simulink model "PF_ParallelHybrid_AllElectric"  (R2021b)
settings: Solver=FixedStepAuto  StartTime=0.0  StopTime=10  FixedStep=0.02  RelTol=1e-3
libraries: Lib_EMTAT x6, slpidlib x1
settings Model: Creator=sbianco1  LastModifiedBy=sbianco1
settings SolverCC: AlgebraicLoopSolver=TrustRegion
settings DebuggingCC: SFMachineParentedDataDiag=warning

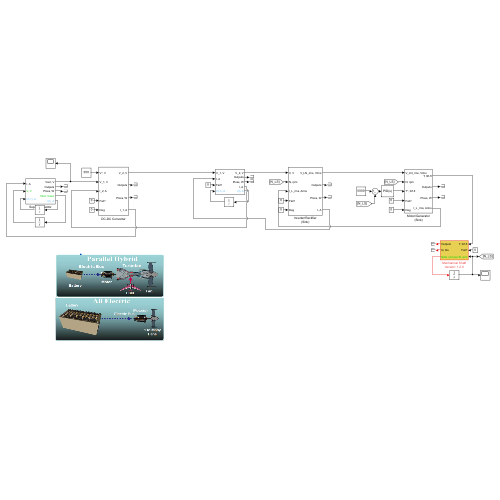
[thumbnail: Simulink's stored preview of the top-level diagram]
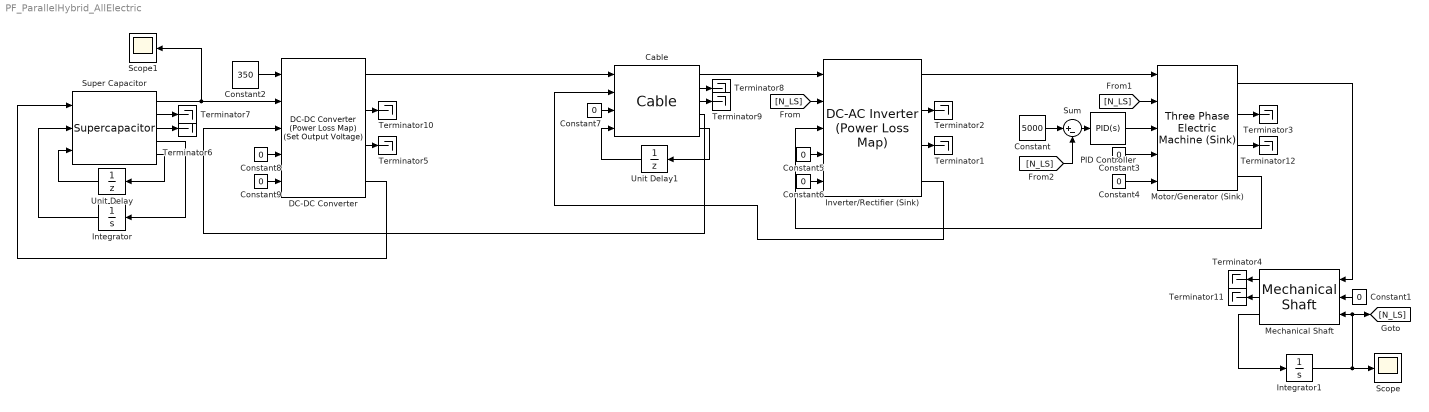
== system PF_ParallelHybrid_AllElectric ==
  Cable : Lib_EMTAT/Components/Power Flow/Cable  R=0.2
  Constant : Constant  Value=5000
  Constant{1,3..9} (8 alike) : Constant  Value=0
  Constant2 : Constant  Value=350
  DC-DC Converter : Lib_EMTAT/Components/Power Flow/DC-DC Converter (Power Loss Map) (Set Output Voltage)  X_Vin_VoltageVec_M=[0 100 1000 5000]  Y_Iout_CurrentVec_M=[0 10 100 150]  T_C_PlossArray_M=100*ones(4,4)  FM=0  Plosslim=0
  Integrator : Integrator  InitialCondition=150
  Integrator1 : Integrator  InitialCondition=5000
  Inverter/Rectifier (Sink) : Lib_EMTAT/Components/Power Flow/DC-AC Inverter (Power Loss Map)  X_C_VoltageInVec_M=[0 1000]  Y_C_RMSCurrentOutVec_M=[0 1000]  T_C_PowLossArray_M=100*ones(2)  K_e=0.0503  FM=0  Plosslim=0
  Mechanical Shaft : Lib_EMTAT/Components/Power Flow/Mechanical Shaft  J=0.01  B=0.001
      settings: AttributesFormatString=|
      | Mechanical Shaft
      | Version: %<LibraryVersion>
  Motor/Generator (Sink) : Lib_EMTAT/Components/Power Flow/Three Phase Electric Machine (Sink)  X_C_SpeedVec_M=[0 100 1000 5000]  Y_C_TorqueVec_M=[0 10 100 150]  T_C_EffArray_M=0.99*ones(4,4)  FM=0
  PID Controller : slpidlib/PID Controller  Controller=PID  Form=Parallel  TimeDomain=Continuous-time  UseExternalTs=off  SampleTime=-1  IntegratorMethod=Forward Euler  FilterMethod=Forward Euler  ControllerParametersSource=internal  P=0.01  I=0.01  D=0  N=100  UseFilter=on  TunerSelectOption=Transfer Function Based (PID Tuner App)  InitialConditionSource=internal  InitialConditionForIntegrator=0  InitialConditionForFilter=0  DifferentiatorICPrevScaledInput=0  ExternalReset=none  TrackingMode=off  Kt=1  LimitOutput=off  SatLimitsSource=internal  UpperSaturationLimit=inf  LowerSaturationLimit=-inf  LinearizeAsGain=on  AntiWindupMode=none  Kb=1  POutMin=[]  POutMax=[]  IOutMin=[]  IOutMax=[]  DOutMin=[]  DOutMax=[]  NOutMin=[]  NOutMax=[]  SumOutMin=[]  SumOutMax=[]  SaturationOutMin=[]  SaturationOutMax=[]  PParamMin=[]  PParamMax=[]  IParamMin=[]  IParamMax=[]  DParamMin=[]  DParamMax=[]  NParamMin=[]  NParamMax=[]  KbParamMin=[]  KbParamMax=[]  KtParamMin=[]  KtParamMax=[]  KbOutMin=[]  KbOutMax=[]  KtOutMin=[]  KtOutMax=[]  IntegratorOutMin=[]  IntegratorOutMax=[]  FilterOutMin=[]  FilterOutMax=[]  SumI1OutMin=[]  SumI1OutMax=[]  SumI2OutMin=[]  SumI2OutMax=[]  SumI3OutMin=[]  SumI3OutMax=[]  SumI4OutMin=[]  SumI4OutMax=[]  SumDOutMin=[]  SumDOutMax=[]  DifferentiatorOutMin=[]  DifferentiatorOutMax=[]  FilterDiffOutCoefMin=[]  FilterDiffOutCoefMax=[]  ReciprocalOutMin=[]  ReciprocalOutMax=[]  SumDenOutMin=[]  SumDenOutMax=[]  SumNumOutMin=[]  SumNumOutMax=[]  DivideOutMin=[]  DivideOutMax=[]  UdiffTsProdOutMin=[]  UdiffTsProdOutMax=[]  NTsProdOutMin=[]  NTsProdOutMax=[]  UintegralTsProdOutMin=[]  UintegralTsProdOutMax=[]  UngainTsProdOutMin=[]  UngainTsProdOutMax=[]  IntegratorContinuousStateAttributes=''  IntegratorStateMustResolveToSignalObject=off  IntegratorRTWStateStorageClass=Auto  FilterContinuousStateAttributes=''  FilterStateMustResolveToSignalObject=off  FilterRTWStateStorageClass=Auto  ParallelPVariant=InternalParameters  IdealPVariant=Disabled  IVariant=InternalParameters  DVariant=InternalParameters  IntegratorVariant=Continuous  SatVariant=Disabled  AWVariant=Passthrough  PCopyVariant=Disabled  TRVariant=Disabled  FdbkBlocksVariant=Forward  IdealPFdbkVariant=Disabled  SatFdbkVariant=Disabled  DerivativeFilterVariant=ContFilter  NVariant=InternalParameters  NCopyVariant=Disabled  FilterICVariant=InternalICsFilter  IntegratorICVariant=InternalICs  ExternalResetVariant=Disabled  TRSumVariant=Passthrough  SumFdbkVariant=Disabled  SumVariant=Sum_PID  TsampFilterVariant=InternalTs  TsampNgainVariant=Passthrough  TsampIntegralVariant=Passthrough  ExternalSaturationOutDataTypeStr=Inherit: Same as second input
  Scope : Scope
  Scope1 : Scope
  Sum : Sum  Inputs=|+-
  Super Capacitor : Lib_EMTAT/Components/Power Flow/Supercapacitor  C=130  ESR=0.02  TSE=200  BlkNm=double(gcb)
  Terminator{1..12} (12 alike) : Terminator
  Unit Delay : UnitDelay  SampleTime=-1  HasFrameUpgradeWarning=on
  Unit Delay1 : UnitDelay  SampleTime=-1  HasFrameUpgradeWarning=on
  wires:
  Inverter/Rectifier (Sink)/1 -> Motor/Generator (Sink)/1
  Constant2/1 -> DC-DC Converter/1
  Super Capacitor/1 -> Scope1/1, DC-DC Converter/2
  Cable/1 -> Inverter/Rectifier (Sink)/1
  Inverter/Rectifier (Sink)/4 -> Cable/2
  Motor/Generator (Sink)/4 -> Inverter/Rectifier (Sink)/3
  [N_LS] -> Inverter/Rectifier (Sink)/2
  [N_LS] -> Motor/Generator (Sink)/2
  Motor/Generator (Sink)/1 -> Mechanical Shaft/1
  Inverter/Rectifier (Sink)/3 -> Terminator1/1
  Inverter/Rectifier (Sink)/2 -> Terminator2/1
  Motor/Generator (Sink)/2 -> Terminator3/1
  DC-DC Converter/4 -> Super Capacitor/1
  Cable/4 -> DC-DC Converter/3
  Super Capacitor/3 -> Terminator6/1
  Super Capacitor/2 -> Terminator7/1
  DC-DC Converter/1 -> Cable/1
  Cable/2 -> Terminator8/1
  Cable/3 -> Terminator9/1
  [N_LS] -> Sum/2
  Sum/1 -> PID Controller/1
  Constant/1 -> Sum/1
  PID Controller/1 -> Motor/Generator (Sink)/3
  DC-DC Converter/3 -> Terminator5/1
  DC-DC Converter/2 -> Terminator10/1
  Super Capacitor/5 -> Unit Delay/1
  Unit Delay/1 -> Super Capacitor/3
  Integrator/1 -> Super Capacitor/2
  Super Capacitor/4 -> Integrator/1
  Cable/5 -> Unit Delay1/1
  Unit Delay1/1 -> Cable/4
  Integrator1/1 -> Scope/1, [N_LS], Mechanical Shaft/3
  Constant1/1 -> Mechanical Shaft/2
  Motor/Generator (Sink)/3 -> Terminator12/1
  Constant3/1 -> Motor/Generator (Sink)/4
  Constant4/1 -> Motor/Generator (Sink)/5
  Constant5/1 -> Inverter/Rectifier (Sink)/4
  Constant6/1 -> Inverter/Rectifier (Sink)/5
  Constant7/1 -> Cable/3
  Constant8/1 -> DC-DC Converter/4
  Constant9/1 -> DC-DC Converter/5
  Mechanical Shaft/1 -> Terminator4/1
  Mechanical Shaft/2 -> Terminator11/1
  Mechanical Shaft/3 -> Integrator1/1
